simulink model "Schema_Bloc_Complet"  (R2015a)
settings: Solver=ode45  StartTime=0.0  StopTime=2  MaxStep=0.0001  RelTol=1e-3
settings Model: Creator=Xavier  LastModifiedBy=Xavier

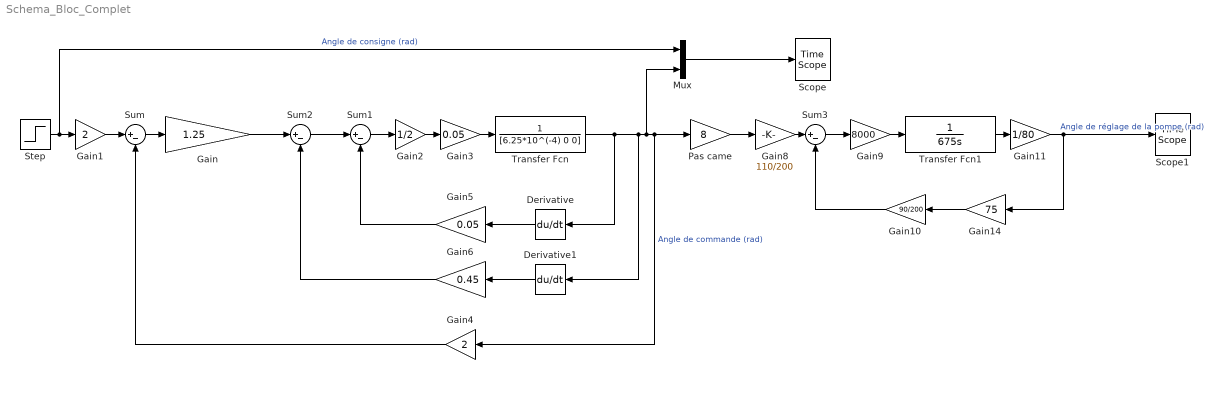
== system Schema_Bloc_Complet ==
  Derivative : Derivative
  Derivative1 : Derivative
  Gain : Gain  Gain=1.25
  Gain1 : Gain  Gain=2
  Gain10 : Gain  Gain=90/200
  Gain11 : Gain  Gain=1/80
  Gain14 : Gain  Gain=75
  Gain2 : Gain  Gain=1/2
  Gain3 : Gain  Gain=0.05
  Gain4 : Gain  Gain=2
  Gain5 : Gain  Gain=0.05
  Gain6 : Gain  Gain=0.45
  Gain8 : Gain  Gain=110/200
  Gain9 : Gain  Gain=8000
  Mux : Mux  Inputs=2
  Pas came : Gain  Gain=8
  Scope : TimeScope
  Scope1 : TimeScope
  Step : Step  Time=0  SampleTime=0
  Sum{,1..3} (4 alike) : Sum  Inputs=|+-
  Transfer Fcn : TransferFcn  Denominator=[6.25*10^(-4) 0 0]
  Transfer Fcn1 : TransferFcn  Denominator=[675 0]
  wires:
  Sum/1 -> Gain/1
  Gain1/1 -> Sum/1
  Sum1/1 -> Gain2/1
  Gain2/1 -> Gain3/1
  Gain3/1 -> Transfer Fcn/1
  Transfer Fcn/1 -> Derivative/1, Derivative1/1, Pas came/1, Gain4/1, Mux/2  "Angle de commande (rad)"
  Gain5/1 -> Sum1/2
  Gain4/1 -> Sum/2
  Derivative/1 -> Gain5/1
  Sum2/1 -> Sum1/1
  Gain/1 -> Sum2/1
  Gain6/1 -> Sum2/2
  Derivative1/1 -> Gain6/1
  Step/1 -> Mux/1, Gain1/1  "Angle de consigne (rad)"
  Mux/1 -> Scope/1
  Gain8/1 -> Sum3/1
  Pas came/1 -> Gain8/1
  Sum3/1 -> Gain9/1
  Gain9/1 -> Transfer Fcn1/1
  Gain11/1 -> Gain14/1, Scope1/1  "Angle de réglage de la pompe (rad)"
  Gain14/1 -> Gain10/1
  Transfer Fcn1/1 -> Gain11/1
  Gain10/1 -> Sum3/2
